simulink model "untitled1"  (R2015a)
settings: Solver=ode45  StartTime=0.0  StopTime=1  RelTol=1e-3
libraries: powerlib x17
settings Model: Creator=MBK  LastModifiedBy=MBK
settings DataIOCC: LimitDataPoints=off

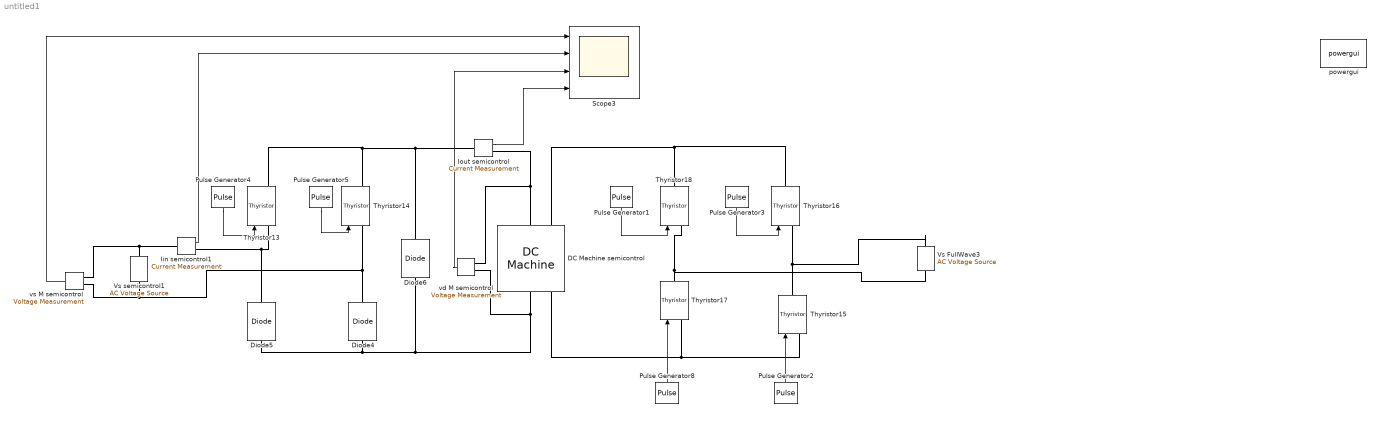
== system untitled1 ==
  DC Machine semicontrol : powerlib/Machines/DC Machine  PresetModel=No  MechanicalLoad=Speed w  FieldType=Wound  ShowDetailedParameters=on  MeasurementBus=off  RLa="[ 0.6  0.12]"  RLf="[ 240  120]"  Laf=1.8  MachineConstant=Torque constant (N.m/A)  Ke=1.8  Kt=1.8  J=1  Bm=0  Tf=0  w0=1  Ifinit=1  TsPowergui=0  TsBlock=-1
  Diode4 : powerlib/Power Electronics/Diode  Ron=0.001  Lon=0  Vf=0.8  IC=0  UseSnubber=off  Rs=500  Cs=250e-9  Measurements=off
  Diode5 : powerlib/Power Electronics/Diode  Ron=0.001  Lon=0  Vf=0.8  IC=0  UseSnubber=off  Rs=500  Cs=250e-9  Measurements=off
  Diode6 : powerlib/Power Electronics/Diode  Ron=0.001  Lon=0  Vf=0.8  IC=0  UseSnubber=off  Rs=500  Cs=250e-9  Measurements=off
  Iin semicontrol1 : powerlib/Measurements/Current Measurement  PhasorSimulation=off  OutputType=Complex  PSBequivalent=0
  Iout semicontrol : powerlib/Measurements/Current Measurement  PhasorSimulation=off  OutputType=Complex  PSBequivalent=0
  Pulse Generator1 : DiscretePulseGenerator  PulseType=Time based  Amplitude=5  Period=0.02  PulseWidth=5  PhaseDelay=60*0.02/360
  Pulse Generator2 : DiscretePulseGenerator  PulseType=Time based  Amplitude=5  Period=0.02  PulseWidth=5  PhaseDelay=60*0.02/360
  Pulse Generator3 : DiscretePulseGenerator  PulseType=Time based  Amplitude=5  Period=0.02  PulseWidth=5  PhaseDelay=240*0.02/360
  Pulse Generator4 : DiscretePulseGenerator  PulseType=Time based  Amplitude=5  Period=0.02  PulseWidth=5  PhaseDelay=60*0.02/360
  Pulse Generator5 : DiscretePulseGenerator  PulseType=Time based  Amplitude=5  Period=0.02  PulseWidth=5  PhaseDelay=240*0.02/360
  Pulse Generator8 : DiscretePulseGenerator  PulseType=Time based  Amplitude=5  Period=0.02  PulseWidth=5  PhaseDelay=240*0.02/360
  Scope3 : Scope  NumInputPorts=4
      settings: YMin=-5~-5~-5~-5  YMax=5~5~5~5  SaveName=ScopeData2
  Thyristor13 : powerlib/Power Electronics/Thyristor  Ron=0.001  Lon=0  Vf=0.8  IC=0  Rs=500  Cs=250e-9  Measurements=on
  Thyristor14 : powerlib/Power Electronics/Thyristor  Ron=0.001  Lon=0  Vf=0.8  IC=0  Rs=500  Cs=250e-9  Measurements=on
  Thyristor{15..18} (4 alike) : powerlib/Power Electronics/Thyristor  Ron=0.001  Lon=0  Vf=0.8  IC=0  Rs=500  Cs=250e-9  Measurements=off
  Vs FullWave3 : powerlib/Electrical Sources/AC Voltage Source  Amplitude=220*sqrt(2)  Phase=0  Frequency=50  SampleTime=0  Measurements=None
  Vs semicontrol1 : powerlib/Electrical Sources/AC Voltage Source  Amplitude=220*sqrt(2)  Phase=0  Frequency=50  SampleTime=0  Measurements=None
  powergui : powerlib/powergui  Priority=1  SimulationMode=Continuous  SolverType=Tustin/Backward Euler (TBE)  SampleTime=50e-6  frequency=60  SPID=off  DisableSnubberDevices=off  DisableRonSwitches=off  DisableVfSwitches=off  SwTol=0  DisplayEquations=off  Interpol=off  methode=off  Ts=100  FunctionMessages=off  echomessages=off  HookPort=off  EnableUseOfTLC=off  x0status=blocks  frequencyindice=0  Pbase=100e6  ErrMax=1e-4  Iterations=50  UnitsV=kV  UnitsW=MW  buscounter=0  RestoreLinks=warning  ResistiveCurrentMeasurement=off  Frange=[0:2:500]  Ylog=off  Xlog=on  ShowGrid=off  save=off  variable=ZData  structure=0  ZoomFFT=off  StartTime=0.0  cycles=1  DisplayStyle=1  fundamental=60  FreqAxis=off  MaxFrequency=1000  frequencyindicesteady=1  RmsSteady=1  display=off
  vd M semicontrol : powerlib/Measurements/Voltage Measurement  PhasorSimulation=off  OutputType=Complex  PSBequivalent=0
  vs M semicontrol : powerlib/Measurements/Voltage Measurement  PhasorSimulation=off  OutputType=Complex  PSBequivalent=0
  wires:
  Pulse Generator2/1 -> Thyristor15/1
  Pulse Generator8/1 -> Thyristor17/1
  vs M semicontrol/1 -> Scope3/1
  Iin semicontrol1/1 -> Scope3/2
  vd M semicontrol/1 -> Scope3/3
  Iout semicontrol/1 -> Scope3/4
  Pulse Generator4/1 -> Thyristor13/1
  Pulse Generator5/1 -> Thyristor14/1
  Pulse Generator1/1 -> Thyristor18/1
  Pulse Generator3/1 -> Thyristor16/1
  connections:
  Diode6/RConn1 -- Iout semicontrol/LConn1 -- Thyristor13/RConn1 -- Thyristor14/RConn1
  vs M semicontrol/LConn2 -- Vs semicontrol1/LConn1 -- Thyristor14/LConn1 -- Diode4/RConn1
  Thyristor15/RConn1 -- Vs FullWave3/RConn1 -- Thyristor16/LConn1
  Thyristor17/RConn1 -- Thyristor18/LConn1 -- Vs FullWave3/LConn1
  Thyristor16/RConn1 -- DC Machine semicontrol/LConn2 -- Thyristor18/RConn1
  Thyristor15/LConn1 -- DC Machine semicontrol/RConn2 -- Thyristor17/LConn1
  DC Machine semicontrol/LConn1 -- vd M semicontrol/LConn1 -- Iout semicontrol/RConn1
  Diode5/RConn1 -- Thyristor13/LConn1 -- Iin semicontrol1/RConn1
  vd M semicontrol/LConn2 -- DC Machine semicontrol/RConn1 -- Diode6/LConn1 -- Diode5/LConn1 -- Diode4/LConn1
  Vs semicontrol1/RConn1 -- vs M semicontrol/LConn1 -- Iin semicontrol1/LConn1
